simulink library "SUB_ECU_L4_MABX_HW_Interface"  (R2018a)
settings: Solver=VariableStepAuto  StartTime=0.0  StopTime=10.0  RelTol=1e-3
PostLoadFcn:
  | , if any(exist('dsrtsu_mdlpostloadfcn', 'file') == [2, 3, 6]), try dsrtsu_mdlpostloadfcn('Execute', bdroot); catch fprintf('Error in PostLoadFcn (dsrtsu_mdlpostloadfcn) for model "%s":\n %s\n', bdroot, lasterr); end, end,
undefined symbols (not defined in the file or in its folder): CANR_PROPB_REAX_3_13_CHANNEL_APV, CANR_PROPB_REAX_4_13_CHANNEL_APV, CANR_PROPB_XPR_1_50_CHANNEL_APV, ENUM_CAN_RX_T, ENUM_CAN_TX_T, ENUM_REAX_OPERATION_MODE_T, ENUM_SIGNAL_HEALTH_T, ENUM_XBR_CONTROL_MODE_T, ENUM_XBR_EBI_MODE_T, ENUM_XBR_PASS_THROUGH_ACTIVE_T, ENUM_XBR_PRIORITY_T, ENUM_XPR_INHIBIT_PARK_MANUAL_T, ENUM_XPR_INHIBIT_UNPARK_MANUAL_T, ENUM_XPR_PARK_MANUAL_T, ENUM_XPR_UNPARK_MANUAL_T, PROPB_REAX_1_E4_DES_POS_SIG_SRC_APV, PROPB_REAX_1_E4_DESIRED_OPMODE_APV, PROPB_REAX_1_E4_DESIRED_POSITION_APV, ptc_matlab_lib
libraries: PTC_MBDS_LIB x264, rtican x172, EmE_MBD_Blockset x39, simulink x34, $bdroot x16, rti1401lib_dio_type4 x8, simulink_need_slupdate x7, dsa_tcpip_lib x4, rti1401lib_adc_type4 x3, rtmapslib x3, rtitasklib x3
(part 13 of 51)

== system SUB_ECU_L4_MABX_HW_Interface/CAN_PIC_KW/CAN_RX_Bendix_RADAR_Tracks/RX_CAN_1 ==
  Enable : Inport
  Bus Creator : BusCreator  Inputs=74
  Data Type Conversion10 : DataTypeConversion  OutDataTypeStr=double  SaturateOnIntegerOverflow=on
  Data Type Conversion8 : DataTypeConversion  OutDataTypeStr=boolean  SaturateOnIntegerOverflow=on
  Data Type Conversion9 : DataTypeConversion  OutDataTypeStr=double  SaturateOnIntegerOverflow=on
  Tracks : rtican/RTICAN Receive (RX)   Reserved1=[]  Reserved2=[]  Reserved3=[]  Reserved4=[]  SfcnMessage=[]  Msg_Struct=[]  BoardTypeNo=[]  BoardNo=[]  ChannelNo=[]  Parameters=[]  DialogFcn=[]  UnitName=[]  Revision=[]  UnitValues=[]  DSProperties=struct('RTI',struct('Version',uint32(5),'BlockType',struct('isSLSource',uint8(1),'isSLSink',uint8(1),'isHWSource',uint8(0),'isHWSink',uint8(0),'isSetup',uint8(0),'isInline',uint8(1),'isNonInline',uint8(0),'isInterrupt',uint8(0),'isChannelwise',uint8(0)),'IOBoardType','RTICAN','UnitType','MESSAGE','Identifier','RX','DialogType','MSVC','BlockSet','RTICAN','SlaveProcessor','CAN'))  RTIBlockInterface=struct('OutputPortsWidth',int32([1 1 1 1 1 1 1 1 1 1 1 1 1 1 1 1 1 1 1 1 1 1 1 1 1 1 1 1 1 1 1 1 1 1 1 1 1 1 1 1 1 1 1 1 1 1 1 1 1 1 1 1 1 1 1 1 1 1 1 1 1 1 1 1 1 1 1 1 1 1 1 1 1 1]),'OutputPortsActive',ones(1,74),'OutputPortsName',{{'tr0_track_selection_status','tr0_corrected_lateral_distance','tr1_track_selection_status','tr1_corrected_lateral_distance','tr2_track_selection_status','tr2_corrected_lateral_distance','tr3_track_selection_status','tr3_corrected_lateral_distance','tr4_track_selection_status','tr4_corrected_lateral_distance','tr5_track_selection_status','tr5_corrected_lateral_distance','tr6_track_selection_status','tr6_corrected_lateral_distance','tr7_track_selection_status','tr7_corrected_lateral_distance','tr8_track_selection_status','tr8_corrected_lateral_distance','tr9_track_selection_status','tr9_corrected_lateral_distance','tr0_lateral_position','tr1_lateral_position','tr2_lateral_position','tr3_lateral_position','tr4_lateral_position','tr5_lateral_position','tr6_lateral_position','tr7_lateral_position','tr8_lateral_position','tr9_lateral_position','tr0_range','tr1_range','tr2_range','tr3_range','tr4_range','tr5_range','tr6_range','tr7_range','tr8_range','tr9_range','tr0_radar_confidence','tr1_radar_confidence','tr2_radar_confidence','tr3_radar_confidence','tr4_radar_confidence','tr5_radar_confidence','tr6_radar_confidence','tr7_radar_confidence','tr8_radar_confidence','tr9_radar_confidence','tr0_relative_velocitiy','tr0_acceleration_over_ground','tr1_relative_velocitiy','tr1_acceleration_over_ground','tr2_relative_velocitiy','tr2_acceleration_over_ground','tr3_relative_velocitiy','tr3_acceleration_over_ground','tr4_relative_velocitiy','tr4_acceleration_over_ground','tr5_relative_velocitiy','tr5_acceleration_over_ground','tr6_relative_velocitiy','tr6_acceleration_over_ground','tr7_relative_velocitiy','tr7_acceleration_over_ground','tr8_relative_velocitiy','tr8_acceleration_over_ground','tr9_relative_velocitiy','tr9_acceleration_over_ground','track_multiplexor',['RX status'],['RX time'],['RX delta time']}},'OutputPortsDataType',{{'SS_DOUBLE','SS_DOUBLE','SS_DOUBLE','SS_DOUBLE','SS_DOUBLE','SS_DOUBLE','SS_DOUBLE','SS_DOUBLE','SS_DOUBLE','SS_DOUBLE','SS_DOUBLE','SS_DOUBLE','SS_DOUBLE','SS_DOUBLE','SS_DOUBLE','SS_DOUBLE','SS_DOUBLE','SS_DOUBLE','SS_DOUBLE','SS_DOUBLE','SS_DOUBLE','SS_DOUBLE','SS_DOUBLE','SS_DOUBLE','SS_DOUBLE','SS_DOUBLE','SS_DOUBLE','SS_DOUBLE','SS_DOUBLE','SS_DOUBLE','SS_DOUBLE','SS_DOUBLE','SS_DOUBLE','SS_DOUBLE','SS_DOUBLE','SS_DOUBLE','SS_DOUBLE','SS_DOUBLE','SS_DOUBLE','SS_DOUBLE','SS_DOUBLE','SS_DOUBLE','SS_DOUBLE','SS_DOUBLE','SS_DOUBLE','SS_DOUBLE','SS_DOUBLE','SS_DOUBLE','SS_DOUBLE','SS_DOUBLE','SS_DOUBLE','SS_DOUBLE','SS_DOUBLE','SS_DOUBLE','SS_DOUBLE','SS_DOUBLE','SS_DOUBLE','SS_DOUBLE','SS_DOUBLE','SS_DOUBLE','SS_DOUBLE','SS_DOUBLE','SS_DOUBLE','SS_DOUBLE','SS_DOUBLE','SS_DOUBLE','SS_DOUBLE','SS_DOUBLE','SS_DOUBLE','SS_DOUBLE','SS_DOUBLE','SS_DOUBLE','SS_DOUBLE','SS_DOUBLE'}},'OutputPortsLabel',{{'tr0_track_selection_status','tr0_corrected_lateral_distance','tr1_track_selection_status','tr1_corrected_lateral_distance','tr2_track_selection_status','tr2_corrected_lateral_distance','tr3_track_selection_status','tr3_corrected_lateral_distance','tr4_track_selection_status','tr4_corrected_lateral_distance','tr5_track_selection_status','tr5_corrected_lateral_distance','tr6_track_selection_status','tr6_corrected_lateral_distance','tr7_track_selection_status','tr7_corrected_lateral_distance','tr8_track_selection_status','tr8_corrected_lateral_distance','tr9_track_selection_status','tr9_corrected_lateral_distance','tr0_lateral_position','tr1_lateral_position','tr2_lateral_position','tr3_lateral_position','tr4_lateral_position','tr5_lateral_position','tr6_lateral_position','tr7_lateral_position','tr8_lateral_position','tr9_lateral_position','tr0_range','tr1_range','tr2_range','tr3_range','tr4_range','tr5_range','tr6_range','tr7_range','tr8_range','tr9_range','tr0_radar_confidence','tr1_radar_confidence','tr2_radar_confidence','tr3_radar_confidence','tr4_radar_confidence','tr5_radar_confidence','tr6_radar_confidence','tr7_radar_confidence','tr8_radar_confidence','tr9_radar_confidence','tr0_relative_velocitiy','tr0_acceleration_over_ground','tr1_relative_velocitiy','tr1_acceleration_over_ground','tr2_relative_velocitiy','tr2_acceleration_over_ground','tr3_relative_velocitiy','tr3_acceleration_over_ground','tr4_relative_velocitiy','tr4_acceleration_over_ground','tr5_relative_velocitiy','tr5_acceleration_over_ground','tr6_relative_velocitiy','tr6_acceleration_over_ground','tr7_relative_velocitiy','tr7_acceleration_over_ground','tr8_relative_velocitiy','tr8_acceleration_over_ground','tr9_relative_velocitiy','tr9_acceleration_over_ground','track_multiplexor','','',''}},'OutputPortsLabelMode','ON','InputPortsWidth',int32(0),'InputPortsActive',0,'DialogFcn','rtican_message_interface_gui','BlockDisplay',{{'','center'}},'IconTransparency','on','ParameterTunableNames',{{}},'InitLevel',3,'BlockName',struct('Token',{{'Tracks'}}),'SampleTime',{{-1}},'TriggerPort',{{'none'}},'EnablePort',{{'yes'}})  RTIBlockParameters=struct('BoardTypeNo',{{1,'OFF',[]}},'BoardNo',{{2,'ON',[1 16]}},'ChannelNo',{{1,'ON',[1 2]}},'Parameters',{{struct('DataFileSupport',struct('DataFileSelectedMaster',1,'DataFileSelectedLocal',0,'DataFileName','c:\data\svn\truck1571\dbc\y257766_004_das_camera_objects_bendix_confidential.dbc|c:\data\svn\truck1571\dbc\y257766_004_das_radar_objects_bendix_confidential.dbc|','DataFileDate',{{{['31-Jan-2018 07:14:07']},{['31-Jan-2018 07:14:07']}}},'SelectedFile','dbc\y257766_004_das_radar_objects_bendix_confidential.dbc'),'Options',struct('StatusSelected',1,'TimeSelected',1,'DeltaTimeSelected',1,'BytePortSelected',0,'MessageLengthSelected',0,'TriggerPort',struct('Selected',0,'TriggerType',0),'UserCoding',struct('Selected',0,'InterfaceFile','UserDecodingFile','FcnName','UserDecodeFcn','InportSelected',0,'InportWidth',1,'OutportSelected',0,'OutportWidth',1),'EnablePortSelected',1,'SignalOnPortnameSelected',1,'UseRXService',1),'Message',struct('MsgOnBlocknameSelected',1,'MsgName','Tracks','MsgIdFormat',0,'MsgId',1635,'MsgLength',8,'NumSignals',71,'SampleTime',-1,'Signal',struct('SgnName',{'tr0_track_selection_status','tr0_corrected_lateral_distance','tr1_track_selection_status','tr1_corrected_lateral_distance','tr2_track_selection_status','tr2_corrected_lateral_distance','tr3_track_selection_status','tr3_corrected_lateral_distance','tr4_track_selection_status','tr4_corrected_lateral_distance','tr5_track_selection_status','tr5_corrected_lateral_distance','tr6_track_selection_status','tr6_corrected_lateral_distance','tr7_track_selection_status','tr7_corrected_lateral_distance','tr8_track_selection_status','tr8_corrected_lateral_distance','tr9_track_selection_status','tr9_corrected_lateral_distance','tr0_lateral_position','tr1_lateral_position','tr2_lateral_position','tr3_lateral_position','tr4_lateral_position','tr5_lateral_position','tr6_lateral_position','tr7_lateral_position','tr8_lateral_position','tr9_lateral_position','tr0_range','tr1_range','tr2_range','tr3_range','tr4_range','tr5_range','tr6_range','tr7_range','tr8_range','tr9_range','tr0_radar_confidence','tr1_radar_confidence','tr2_radar_confidence','tr3_radar_confidence','tr4_radar_confidence','tr5_radar_confidence','tr6_radar_confidence','tr7_radar_confidence','tr8_radar_confidence','tr9_radar_confidence','tr0_relative_velocitiy','tr0_acceleration_over_ground','tr1_relative_velocitiy','tr1_acceleration_over_ground','tr2_relative_velocitiy','tr2_acceleration_over_ground','tr3_relative_velocitiy','tr3_acceleration_over_ground','tr4_relative_velocitiy','tr4_acceleration_over_ground','tr5_relative_velocitiy','tr5_acceleration_over_ground','tr6_relative_velocitiy','tr6_acceleration_over_ground','tr7_relative_velocitiy','tr7_acceleration_over_ground','tr8_relative_velocitiy','tr8_acceleration_over_ground','tr9_relative_velocitiy','tr9_acceleration_over_ground','track_multiplexor'},'SgnStartBit',{0,0,0,0,0,0,0,0,0,0,0,0,0,0,0,0,0,0,0,0,14,14,14,14,14,14,14,14,14,14,16,16,16,16,16,16,16,16,16,16,24,24,24,24,24,24,24,24,24,24,32,32,32,32,32,32,32,32,32,32,32,32,32,32,32,32,32,32,32,32,56},'SgnLength',{13,16,13,16,13,16,13,16,13,16,13,16,13,16,13,16,13,16,13,16,10,10,10,10,10,10,10,10,10,10,16,16,16,16,16,16,16,16,16,16,8,8,8,8,8,8,8,8,8,8,14,8,14,8,14,8,14,8,14,8,14,8,14,8,14,8,14,8,14,8,8},'SgnType',{2,2,2,2,2,2,2,2,2,2,2,2,2,2,2,2,2,2,2,2,2,2,2,2,2,2,2,2,2,2,2,2,2,2,2,2,2,2,2,2,2,2,2,2,2,2,2,2,2,2,2,2,2,2,2,2,2,2,2,2,2,2,2,2,2,2,2,2,2,2,1},'ModeValue',{4,5,12,13,20,21,28,29,36,37,44,45,52,53,60,61,68,69,76,77,6,14,22,30,38,46,54,62,70,78,4,12,20,28,36,44,52,60,68,76,6,14,22,30,38,46,54,62,70,78,4,5,12,13,20,21,28,29,36,37,44,45,52,53,60,61,68,69,76,77,-1},'DataType',{0,1,0,1,0,1,0,1,0,1,0,1,0,1,0,1,0,1,0,1,1,1,1,1,1,1,1,1,1,1,0,0,0,0,0,0,0,0,0,0,0,0,0,0,0,0,0,0,0,0,1,0,1,0,1,0,1,0,1,0,1,0,1,0,1,0,1,0,1,0,0},'ByteLayout',{2,2,2,2,2,2,2,2,2,2,2,2,2,2,2,2,2,2,2,2,2,2,2,2,2,2,2,2,2,2,2,2,2,2,2,2,2,2,2,2,2,2,2,2,2,2,2,2,2,2,2,2,2,2,2,2,2,2,2,2,2,2,2,2,2,2,2,2,2,2,2},'Factor',{1,0.001,1,0.001,1,0.001,1,0.001,1,0.001,1,0.001,1,0.001,1,0.001,1,0.001,1,0.001,0.1,0.1,0.1,0.1,0.1,0.1,0.1,0.1,0.1,0.1,0.01,0.01,0.01,0.01,0.01,0.01,0.01,0.01,0.01,0.01,0.0039215686274509803,0.0039215686274509803,0.0039215686274509803,0.0039215686274509803,0.0039215686274509803,0.0039215686274509803,0.0039215686274509803,0.0039215686274509803,0.0039215686274509803,0.0039215686274509803,0.01,0.05,0.01,0.05,0.01,0.05,0.01,0.05,0.01,0.05,0.01,0.05,0.01,0.05,0.01,0.05,0.01,0.05,0.01,0.05,1},'Offset',{0,0,0,0,0,0,0,0,0,0,0,0,0,0,0,0,0,0,0,0,0,0,0,0,0,0,0,0,0,0,0,0,0,0,0,0,0,0,0,0,0,0,0,0,0,0,0,0,0,0,0,-8.8,0,-8.8,0,-8.8,0,-8.8,0,-8.8,0,-8.8,0,-8.8,0,-8.8,0,-8.8,0,-8.8,0},'SgnComment',{{''},{''},{''},{''},{''},{''},{''},{''},{''},{''},{''},{''},{''},{''},{''},{''},{''},{''},{''},{''},{''},{''},{''},{''},{''},{''},{''},{''},{''},{''},{''},{''},{''},{''},{''},{''},{''},{''},{''},{''},{''},{''},{''},{''},{''},{''},{''},{''},{''},{''},{''},{''},{''},{''},{''},{''},{''},{''},{''},{''},{''},{''},{''},{''},{''},{''},{''},{''},{''},{''},{''}},'SgnUnit',{'','m','','m','','m','','m','','m','','m','','m','','m','','m','','m','m','m','m','m','m','m','m','m','m','m','m','m','m','m','m','m','m','m','m','m','','','','','','','','','','','m/s','m/s²','m/s','m/s²','m/s','m/s²','m/s','m/s²','m/s','m/s²','m/s','m/s²','m/s','m/s²','m/s','m/s²','m/s','m/s²','m/s','m/s²',''},'Min',{0,0,0,0,0,0,0,0,0,0,0,0,0,0,0,0,0,0,0,0,0,0,0,0,0,0,0,0,0,0,0,0,0,0,0,0,0,0,0,0,0,0,0,0,0,0,0,0,0,0,0,0,0,0,0,0,0,0,0,0,0,0,0,0,0,0,0,0,0,0,0},'Max',{0,0,0,0,0,0,0,0,0,0,0,0,0,0,0,0,0,0,0,0,0,0,0,0,0,0,0,0,0,0,0,0,0,0,0,0,0,0,0,0,1,1,1,1,1,1,1,1,1,1,0,0,0,0,0,0,0,0,0,0,0,0,0,0,0,0,0,0,0,0,0},'SLDataType',{'SS_DOUBLE','SS_DOUBLE','SS_DOUBLE','SS_DOUBLE','SS_DOUBLE','SS_DOUBLE','SS_DOUBLE','SS_DOUBLE','SS_DOUBLE','SS_DOUBLE','SS_DOUBLE','SS_DOUBLE','SS_DOUBLE','SS_DOUBLE','SS_DOUBLE','SS_DOUBLE','SS_DOUBLE','SS_DOUBLE','SS_DOUBLE','SS_DOUBLE','SS_DOUBLE','SS_DOUBLE','SS_DOUBLE','SS_DOUBLE','SS_DOUBLE','SS_DOUBLE','SS_DOUBLE','SS_DOUBLE','SS_DOUBLE','SS_DOUBLE','SS_DOUBLE','SS_DOUBLE','SS_DOUBLE','SS_DOUBLE','SS_DOUBLE','SS_DOUBLE','SS_DOUBLE','SS_DOUBLE','SS_DOUBLE','SS_DOUBLE','SS_DOUBLE','SS_DOUBLE','SS_DOUBLE','SS_DOUBLE','SS_DOUBLE','SS_DOUBLE','SS_DOUBLE','SS_DOUBLE','SS_DOUBLE','SS_DOUBLE','SS_DOUBLE','SS_DOUBLE','SS_DOUBLE','SS_DOUBLE','SS_DOUBLE','SS_DOUBLE','SS_DOUBLE','SS_DOUBLE','SS_DOUBLE','SS_DOUBLE','SS_DOUBLE','SS_DOUBLE','SS_DOUBLE','SS_DOUBLE','SS_DOUBLE','SS_DOUBLE','SS_DOUBLE','SS_DOUBLE','SS_DOUBLE','SS_DOUBLE','SS_DOUBLE'}),'MsgIdNumFormat',1,'MsgComment',{{''}}),'Version',1.2,'general',struct('isFromLib',0)),'OFF',[]}},'GroupId',{{struct('Group',{{'RTICAN'}},'No',27,'Behavior',{{'NAMECHANGE'}},'BlockType',{{'SINK'}},'NameChangeFlag',0),'OFF',[]}},'SFcnRTICANMessage',{{struct('MsgType','RX','SFcnPortType','Scalar','MsgName','Tracks','MsgIdFormat','STD','MsgId',1635,'MsgLength',8,'NumSignals',71,'SampleTime',-1,'Signal',struct('SgnName',{'tr0_track_selection_status','tr0_corrected_lateral_distance','tr1_track_selection_status','tr1_corrected_lateral_distance','tr2_track_selection_status','tr2_corrected_lateral_distance','tr3_track_selection_status','tr3_corrected_lateral_distance','tr4_track_selection_status','tr4_corrected_lateral_distance','tr5_track_selection_status','tr5_corrected_lateral_distance','tr6_track_selection_status','tr6_corrected_lateral_distance','tr7_track_selection_status','tr7_corrected_lateral_distance','tr8_track_selection_status','tr8_corrected_lateral_distance','tr9_track_selection_status','tr9_corrected_lateral_distance','tr0_lateral_position','tr1_lateral_position','tr2_lateral_position','tr3_lateral_position','tr4_lateral_position','tr5_lateral_position','tr6_lateral_position','tr7_lateral_position','tr8_lateral_position','tr9_lateral_position','tr0_range','tr1_range','tr2_range','tr3_range','tr4_range','tr5_range','tr6_range','tr7_range','tr8_range','tr9_range','tr0_radar_confidence','tr1_radar_confidence','tr2_radar_confidence','tr3_radar_confidence','tr4_radar_confidence','tr5_radar_confidence','tr6_radar_confidence','tr7_radar_confidence','tr8_radar_confidence','tr9_radar_confidence','tr0_relative_velocitiy','tr0_acceleration_over_ground','tr1_relative_velocitiy','tr1_acceleration_over_ground','tr2_relative_velocitiy','tr2_acceleration_over_ground','tr3_relative_velocitiy','tr3_acceleration_over_ground','tr4_relative_velocitiy','tr4_acceleration_over_ground','tr5_relative_velocitiy','tr5_acceleration_over_ground','tr6_relative_velocitiy','tr6_acceleration_over_ground','tr7_relative_velocitiy','tr7_acceleration_over_ground','tr8_relative_velocitiy','tr8_acceleration_over_ground','tr9_relative_velocitiy','tr9_acceleration_over_ground','track_multiplexor'},'SgnStartBit',{0,0,0,0,0,0,0,0,0,0,0,0,0,0,0,0,0,0,0,0,14,14,14,14,14,14,14,14,14,14,16,16,16,16,16,16,16,16,16,16,24,24,24,24,24,24,24,24,24,24,32,32,32,32,32,32,32,32,32,32,32,32,32,32,32,32,32,32,32,32,56},'SgnLength',{13,16,13,16,13,16,13,16,13,16,13,16,13,16,13,16,13,16,13,16,10,10,10,10,10,10,10,10,10,10,16,16,16,16,16,16,16,16,16,16,8,8,8,8,8,8,8,8,8,8,14,8,14,8,14,8,14,8,14,8,14,8,14,8,14,8,14,8,14,8,8},'SgnType',{'mode-dependent','mode-dependent','mode-dependent','mode-dependent','mode-dependent','mode-dependent','mode-dependent','mode-dependent','mode-dependent','mode-dependent','mode-dependent','mode-dependent','mode-dependent','mode-dependent','mode-dependent','mode-dependent','mode-dependent','mode-dependent','mode-dependent','mode-dependent','mode-dependent','mode-dependent','mode-dependent','mode-dependent','mode-dependent','mode-dependent','mode-dependent','mode-dependent','mode-dependent','mode-dependent','mode-dependent','mode-dependent','mode-dependent','mode-dependent','mode-dependent','mode-dependent','mode-dependent','mode-dependent','mode-dependent','mode-dependent','mode-dependent','mode-dependent','mode-dependent','mode-dependent','mode-dependent','mode-dependent','mode-dependent','mode-dependent','mode-dependent','mode-dependent','mode-dependent','mode-dependent','mode-dependent','mode-dependent','mode-dependent','mode-dependent','mode-dependent','mode-dependent','mode-dependent','mode-dependent','mode-dependent','mode-dependent','mode-dependent','mode-dependent','mode-dependent','mode-dependent','mode-dependent','mode-dependent','mode-dependent','mode-dependent','mode'},'ModeValue',{4,5,12,13,20,21,28,29,36,37,44,45,52,53,60,61,68,69,76,77,6,14,22,30,38,46,54,62,70,78,4,12,20,28,36,44,52,60,68,76,6,14,22,30,38,46,54,62,70,78,4,5,12,13,20,21,28,29,36,37,44,45,52,53,60,61,68,69,76,77,-1},'DataType',{['unsigned int'],['signed int'],['unsigned int'],['signed int'],['unsigned int'],['signed int'],['unsigned int'],['signed int'],['unsigned int'],['signed int'],['unsigned int'],['signed int'],['unsigned int'],['signed int'],['unsigned int'],['signed int'],['unsigned int'],['signed int'],['unsigned int'],['signed int'],['signed int'],['signed int'],['signed int'],['signed int'],['signed int'],['signed int'],['signed int'],['signed int'],['signed int'],['signed int'],['unsigned int'],['unsigned int'],['unsigned int'],['unsigned int'],['unsigned int'],['unsigned int'],['unsigned int'],['unsigned int'],['unsigned int'],['unsigned int'],['unsigned int'],['unsigned int'],['unsigned int'],['unsigned int'],['unsigned int'],['unsigned int'],['unsigned int'],['unsigned int'],['unsigned int'],['unsigned int'],['signed int'],['unsigned int'],['signed int'],['unsigned int'],['signed int'],['unsigned int'],['signed int'],['unsigned int'],['signed int'],['unsigned int'],['signed int'],['unsigned int'],['signed int'],['unsigned int'],['signed int'],['unsigned int'],['signed int'],['unsigned int'],['signed int'],['unsigned int'],['unsigned int']},'ByteLayout',{['motorola back.'],['motorola back.'],['motorola back.'],['motorola back.'],['motorola back.'],['motorola back.'],['motorola back.'],['motorola back.'],['motorola back.'],['motorola back.'],['motorola back.'],['motorola back.'],['motorola back.'],['motorola back.'],['motorola back.'],['motorola back.'],['motorola back.'],['motorola back.'],['motorola back.'],['motorola back.'],['motorola back.'],['motorola back.'],['motorola back.'],['motorola back.'],['motorola back.'],['motorola back.'],['motorola back.'],['motorola back.'],['motorola back.'],['motorola back.'],['motorola back.'],['motorola back.'],['motorola back.'],['motorola back.'],['motorola back.'],['motorola back.'],['motorola back.'],['motorola back.'],['motorola back.'],['motorola back.'],['motorola back.'],['motorola back.'],['motorola back.'],['motorola back.'],['motorola back.'],['motorola back.'],['motorola back.'],['motorola back.'],['motorola back.'],['motorola back.'],['motorola back.'],['motorola back.'],['motorola back.'],['motorola back.'],['motorola back.'],['motorola back.'],['motorola back.'],['motorola back.'],['motorola back.'],['motorola back.'],['motorola back.'],['motorola back.'],['motorola back.'],['motorola back.'],['motorola back.'],['motorola back.'],['motorola back.'],['motorola back.'],['motorola back.'],['motorola back.'],['motorola back.']},'Factor',{1,0.001,1,0.001,1,0.001,1,0.001,1,0.001,1,0.001,1,0.001,1,0.001,1,0.001,1,0.001,0.1,0.1,0.1,0.1,0.1,0.1,0.1,0.1,0.1,0.1,0.01,0.01,0.01,0.01,0.01,0.01,0.01,0.01,0.01,0.01,0.0039215686274509803,0.0039215686274509803,0.0039215686274509803,0.0039215686274509803,0.0039215686274509803,0.0039215686274509803,0.0039215686274509803,0.0039215686274509803,0.0039215686274509803,0.0039215686274509803,0.01,0.05,0.01,0.05,0.01,0.05,0.01,0.05,0.01,0.05,0.01,0.05,0.01,0.05,0.01,0.05,0.01,0.05,0.01,0.05,1},'Offset',{0,0,0,0,0,0,0,0,0,0,0,0,0,0,0,0,0,0,0,0,0,0,0,0,0,0,0,0,0,0,0,0,0,0,0,0,0,0,0,0,0,0,0,0,0,0,0,0,0,0,0,-8.8,0,-8.8,0,-8.8,0,-8.8,0,-8.8,0,-8.8,0,-8.8,0,-8.8,0,-8.8,0,-8.8,0},'SLDataType',{'SS_DOUBLE','SS_DOUBLE','SS_DOUBLE','SS_DOUBLE','SS_DOUBLE','SS_DOUBLE','SS_DOUBLE','SS_DOUBLE','SS_DOUBLE','SS_DOUBLE','SS_DOUBLE','SS_DOUBLE','SS_DOUBLE','SS_DOUBLE','SS_DOUBLE','SS_DOUBLE','SS_DOUBLE','SS_DOUBLE','SS_DOUBLE','SS_DOUBLE','SS_DOUBLE','SS_DOUBLE','SS_DOUBLE','SS_DOUBLE','SS_DOUBLE','SS_DOUBLE','SS_DOUBLE','SS_DOUBLE','SS_DOUBLE','SS_DOUBLE','SS_DOUBLE','SS_DOUBLE','SS_DOUBLE','SS_DOUBLE','SS_DOUBLE','SS_DOUBLE','SS_DOUBLE','SS_DOUBLE','SS_DOUBLE','SS_DOUBLE','SS_DOUBLE','SS_DOUBLE','SS_DOUBLE','SS_DOUBLE','SS_DOUBLE','SS_DOUBLE','SS_DOUBLE','SS_DOUBLE','SS_DOUBLE','SS_DOUBLE','SS_DOUBLE','SS_DOUBLE','SS_DOUBLE','SS_DOUBLE','SS_DOUBLE','SS_DOUBLE','SS_DOUBLE','SS_DOUBLE','SS_DOUBLE','SS_DOUBLE','SS_DOUBLE','SS_DOUBLE','SS_DOUBLE','SS_DOUBLE','SS_DOUBLE','SS_DOUBLE','SS_DOUBLE','SS_DOUBLE','SS_DOUBLE','SS_DOUBLE','SS_DOUBLE'}),'StatusSelected','yes','TimeSelected','yes','DeltaTimeSelected','yes','BytePortSelected','no','MessageLengthSelected','no','TriggerPort',struct('Selected','no','TriggerType',0),'UserCoding',struct('Selected','no','InterfaceFile','UserDecodingFile','FcnName','UserDecodeFcn','InportSelected','no','InportWidth',1,'OutportSelected','no','OutportWidth',1),'EnablePortSelected','yes','UseRXService','yes','BoardType','DS1','BoardNo',2,'ControllerNo',1),'OFF',[]}},'TLCFileName',{{'rtican_rx_message','OFF',[]}})  RTISFcnParameters=struct('SFcnRTICANMessage','struct','TLCFileName','char')  RTIBlockParaDefault=struct('BoardTypeNo',4302,'BoardNo',1,'ChannelNo',1,'Parameters',struct('DataFileSupport',struct('DataFileSelectedMaster',0,'DataFileSelectedLocal',0,'DataFileName','','DataFileDate','','SelectedFile',['<no file selected>']),'Options',struct('StatusSelected',1,'TimeSelected',1,'DeltaTimeSelected',1,'BytePortSelected',0,'MessageLengthSelected',0,'TriggerPort',struct('Selected',0,'TriggerType','rising'),'UserCoding',struct('Selected',0,'InterfaceFile','UserDecodingFile','FcnName','UserDecodeFcn','InportSelected',0,'InportWidth',1,'OutportSelected',0,'OutportWidth',1),'EnablePortSelected',0,'SignalOnPortnameSelected',1,'UseRXService',0),'Message',struct('MsgOnBlocknameSelected',0,'MsgName',['RX Message'],'MsgIdFormat',0,'MsgId',100,'MsgLength',8,'NumSignals',1,'SampleTime',-1,'Signal',struct('SgnName',['RX signal'],'SgnStartBit',0,'SgnLength',8,'SgnType',0,'ModeValue',-1,'DataType',0,'SLDataType','SS_DOUBLE','ByteLayout',0,'Factor',1,'Offset',0,'Min',0,'Max',255,'SgnComment',{{}},'SgnUnit',''),'MsgIdNumFormat',0,'MsgComment',{{''}}),'Version',1.2,'general',struct('isFromLib',1)),'GroupId',struct('Group',{{'RTICAN'}},'No',1,'Behavior',{{'NAMECHANGE'}},'BlockType',{{'SINK'}},'NameChangeFlag',0),'SFcnRTICANMessage',struct('MsgType','RX','MsgName',['RX Message'],'MsgIdFormat','STD','MsgId',100,'MsgLength',8,'NumSignals',1,'SampleTime',-1,'Signal',struct('SgnName',['RX signal'],'SgnStartBit',0,'SgnLength',8,'SgnType','standard','ModeValue',-1,'DataType',['unsigned int'],'ByteLayout',['little endian'],'SLDataType','SS_DOUBLE','Factor',1,'Offset',0),'StatusSelected','yes','TimeSelected','yes','DeltaTimeSelected','yes','BytePortSelected','no','MessageLengthSelected','no','EnablePortSelected','no','UserCoding',struct('Selected','no','InterfaceFile','UserDecodingFile','FcnName','UserDecodeFcn','InportSelected','no','InportWidth',1,'OutportSelected','no','OutportWidth',1),'TriggerPort',struct('Selected','no','TriggerType','rising'),'UseRXService','no','BoardType','DS4302','BoardNo',1,'ControllerNo',1,'SFcnPortType','Scalar'),'TLCFileName','rtican_rx_message')
      settings: AttributesFormatString=Group Id: RTICAN27\n  SourceProductName=dSPACE RTI CAN Blockset
  Bendix_RADAR_Tracks : Outport
  wires:
  Enable/1 -> Tracks/Enable
  Tracks/74 -> Data Type Conversion10/1
  Tracks/73 -> Data Type Conversion9/1
  Tracks/72 -> Data Type Conversion8/1
  Tracks/29 -> Bus Creator/29  "tr8_lateral_position"
  Tracks/28 -> Bus Creator/28  "tr7_lateral_position"
  Tracks/30 -> Bus Creator/30  "tr9_lateral_position"
  Tracks/27 -> Bus Creator/27  "tr6_lateral_position"
  Tracks/31 -> Bus Creator/31  "tr0_range"
  Tracks/26 -> Bus Creator/26  "tr5_lateral_position"
  Tracks/32 -> Bus Creator/32  "tr1_range"
  Tracks/25 -> Bus Creator/25  "tr4_lateral_position"
  Tracks/33 -> Bus Creator/33  "tr2_range"
  Tracks/24 -> Bus Creator/24  "tr3_lateral_position"
  Tracks/34 -> Bus Creator/34  "tr3_range"
  Tracks/23 -> Bus Creator/23  "tr2_lateral_position"
  Tracks/35 -> Bus Creator/35  "tr4_range"
  Tracks/22 -> Bus Creator/22  "tr1_lateral_position"
  Tracks/36 -> Bus Creator/36  "tr5_range"
  Tracks/21 -> Bus Creator/21  "tr0_lateral_position"
  Tracks/37 -> Bus Creator/37  "tr6_range"
  Tracks/20 -> Bus Creator/20  "tr9_corrected_lateral_distance"
  Tracks/38 -> Bus Creator/38  "tr7_range"
  Tracks/19 -> Bus Creator/19  "tr9_track_selection_status"
  Tracks/39 -> Bus Creator/39  "tr8_range"
  Tracks/18 -> Bus Creator/18  "tr8_corrected_lateral_distance"
  Tracks/40 -> Bus Creator/40  "tr9_range"
  Tracks/17 -> Bus Creator/17  "tr8_track_selection_status"
  Tracks/41 -> Bus Creator/41  "tr0_radar_confidence"
  Tracks/16 -> Bus Creator/16  "tr7_corrected_lateral_distance"
  Tracks/42 -> Bus Creator/42  "tr1_radar_confidence"
  Tracks/15 -> Bus Creator/15  "tr7_track_selection_status"
  Tracks/43 -> Bus Creator/43  "tr2_radar_confidence"
  Tracks/14 -> Bus Creator/14  "tr6_corrected_lateral_distance"
  Tracks/44 -> Bus Creator/44  "tr3_radar_confidence"
  Tracks/13 -> Bus Creator/13  "tr6_track_selection_status"
  Tracks/45 -> Bus Creator/45  "tr4_radar_confidence"
  Tracks/12 -> Bus Creator/12  "tr5_corrected_lateral_distance"
  Tracks/46 -> Bus Creator/46  "tr5_radar_confidence"
  Tracks/11 -> Bus Creator/11  "tr5_track_selection_status"
  Tracks/47 -> Bus Creator/47  "tr6_radar_confidence"
  Tracks/10 -> Bus Creator/10  "tr4_corrected_lateral_distance"
  Tracks/48 -> Bus Creator/48  "tr7_radar_confidence"
  Tracks/9 -> Bus Creator/9  "tr4_track_selection_status"
  Tracks/49 -> Bus Creator/49  "tr8_radar_confidence"
  Tracks/8 -> Bus Creator/8  "tr3_corrected_lateral_distance"
  Tracks/50 -> Bus Creator/50  "tr9_radar_confidence"
  Tracks/7 -> Bus Creator/7  "tr3_track_selection_status"
  Tracks/51 -> Bus Creator/51  "tr0_relative_velocitiy"
  Tracks/6 -> Bus Creator/6  "tr2_corrected_lateral_distance"
  Tracks/52 -> Bus Creator/52  "tr0_acceleration_over_ground"
  Tracks/5 -> Bus Creator/5  "tr2_track_selection_status"
  Tracks/53 -> Bus Creator/53  "tr1_relative_velocitiy"
  Tracks/4 -> Bus Creator/4  "tr1_corrected_lateral_distance"
  Tracks/54 -> Bus Creator/54  "tr1_acceleration_over_ground"
  Tracks/3 -> Bus Creator/3  "tr1_track_selection_status"
  Tracks/55 -> Bus Creator/55  "tr2_relative_velocitiy"
  Tracks/2 -> Bus Creator/2  "tr0_corrected_lateral_distance"
  Tracks/56 -> Bus Creator/56  "tr2_acceleration_over_ground"
  Tracks/1 -> Bus Creator/1  "tr0_track_selection_status"
  Tracks/57 -> Bus Creator/57  "tr3_relative_velocitiy"
  Tracks/58 -> Bus Creator/58  "tr3_acceleration_over_ground"
  Tracks/59 -> Bus Creator/59  "tr4_relative_velocitiy"
  Tracks/60 -> Bus Creator/60  "tr4_acceleration_over_ground"
  Tracks/61 -> Bus Creator/61  "tr5_relative_velocitiy"
  Tracks/62 -> Bus Creator/62  "tr5_acceleration_over_ground"
  Tracks/63 -> Bus Creator/63  "tr6_relative_velocitiy"
  Tracks/64 -> Bus Creator/64  "tr6_acceleration_over_ground"
  Tracks/65 -> Bus Creator/65  "tr7_relative_velocitiy"
  Tracks/66 -> Bus Creator/66  "tr7_acceleration_over_ground"
  Tracks/67 -> Bus Creator/67  "tr8_relative_velocitiy"
  Tracks/68 -> Bus Creator/68  "tr8_acceleration_over_ground"
  Tracks/69 -> Bus Creator/69  "tr9_relative_velocitiy"
  Tracks/70 -> Bus Creator/70  "tr9_acceleration_over_ground"
  Tracks/71 -> Bus Creator/71  "track_multiplexor"
  Data Type Conversion8/1 -> Bus Creator/72  "Bendix_RADAR_Tracks_RX_status"
  Data Type Conversion9/1 -> Bus Creator/73  "Bendix_RADAR_Tracks_RX_time"
  Data Type Conversion10/1 -> Bus Creator/74  "Bendix_RADAR_Tracks_RX_delta_time"
  Bus Creator/1 -> Bendix_RADAR_Tracks/1  "Bendix_RADAR_Tracks"

== system SUB_ECU_L4_MABX_HW_Interface/CAN_PIC_KW/CAN_RX_CCVS1_00/RX_CAN_1 ==
  Enable : Inport
  Bus Creator : BusCreator  Inputs=20
  Bus Creator3 : BusCreator  Inputs=4
  CCVS1_00 : rtican/RTICAN Receive (RX)   Reserved1=[]  Reserved2=[]  Reserved3=[]  Reserved4=[]  SfcnMessage=[]  Msg_Struct=[]  BoardTypeNo=[]  BoardNo=[]  ChannelNo=[]  Parameters=[]  DialogFcn=[]  UnitName=[]  Revision=[]  UnitValues=[]  DSProperties=struct('RTI',struct('Version',uint32(5),'BlockType',struct('isSLSource',uint8(1),'isSLSink',uint8(1),'isHWSource',uint8(0),'isHWSink',uint8(0),'isSetup',uint8(0),'isInline',uint8(1),'isNonInline',uint8(0),'isInterrupt',uint8(0),'isChannelwise',uint8(0)),'IOBoardType','RTICAN','UnitType','MESSAGE','Identifier','RX','DialogType','MSVC','BlockSet','RTICAN','SlaveProcessor','CAN'))  RTIBlockInterface=struct('OutputPortsWidth',int32([1 1 1 1 1 1 1 1 1 1 1 1 1 1 1 1 1 1 1 1 1 1 1]),'OutputPortsActive',ones(1,23),'OutputPortsName',{{'TwoSpeedAxleSwitch','ParkingBrakeSwitch','CruiseCtrlPauseSwitch','ParkBrakeReleaseInhibitRq','WheelBasedVehicleSpeed','CruiseCtrlActive','CruiseCtrlEnableSwitch','BrakeSwitch','ClutchSwitch','CruiseCtrlSetSwitch','CruiseCtrlCoastSwitch','CruiseCtrlResumeSwitch','CruiseCtrlAccelerateSwitch','CruiseCtrlSetSpeed','PTOGovernorState','CruiseCtrlStates','EngIdleIncrementSwitch','EngIdleDecrementSwitch','EngTestModeSwitch','EngShutdownOverrideSwitch',['RX status'],['RX time'],['RX delta time']}},'OutputPortsDataType',{{'SS_DOUBLE','SS_DOUBLE','SS_DOUBLE','SS_DOUBLE','SS_DOUBLE','SS_DOUBLE','SS_DOUBLE','SS_DOUBLE','SS_DOUBLE','SS_DOUBLE','SS_DOUBLE','SS_DOUBLE','SS_DOUBLE','SS_DOUBLE','SS_DOUBLE','SS_DOUBLE','SS_DOUBLE','SS_DOUBLE','SS_DOUBLE','SS_DOUBLE','SS_DOUBLE','SS_DOUBLE','SS_DOUBLE'}},'OutputPortsLabel',{{'TwoSpeedAxleSwitch','ParkingBrakeSwitch','CruiseCtrlPauseSwitch','ParkBrakeReleaseInhibitRq','WheelBasedVehicleSpeed','CruiseCtrlActive','CruiseCtrlEnableSwitch','BrakeSwitch','ClutchSwitch','CruiseCtrlSetSwitch','CruiseCtrlCoastSwitch','CruiseCtrlResumeSwitch','CruiseCtrlAccelerateSwitch','CruiseCtrlSetSpeed','PTOGovernorState','CruiseCtrlStates','EngIdleIncrementSwitch','EngIdleDecrementSwitch','EngTestModeSwitch','EngShutdownOverrideSwitch','','',''}},'OutputPortsLabelMode','ON','InputPortsWidth',int32(0),'InputPortsActive',0,'DialogFcn','rtican_message_interface_gui','BlockDisplay',{{'','center'}},'IconTransparency','on','ParameterTunableNames',{{}},'InitLevel',3,'BlockName',struct('Token',{{'CCVS1_00'}}),'SampleTime',{{-1}},'TriggerPort',{{'none'}},'EnablePort',{{'yes'}})  RTIBlockParameters=struct('BoardTypeNo',{{1,'OFF',[]}},'BoardNo',{{1,'ON',[1 16]}},'ChannelNo',{{1,'ON',[1 2]}},'Parameters',{{struct('DataFileSupport',struct('DataFileSelectedMaster',1,'DataFileSelectedLocal',0,'DataFileName','c:\localdata\chris\advanced_tech\adas\level4_rcp\truck1571\dbc\mabx_can1.dbc|','DataFileDate',{{{['03-Apr-2017 12:55:40']}}},'SelectedFile',['<no file selected>']),'Options',struct('StatusSelected',1,'TimeSelected',1,'DeltaTimeSelected',1,'BytePortSelected',0,'MessageLengthSelected',0,'TriggerPort',struct('Selected',0,'TriggerType',0),'UserCoding',struct('Selected',0,'InterfaceFile','UserDecodingFile','FcnName','UserDecodeFcn','InportSelected',0,'InportWidth',1,'OutportSelected',0,'OutportWidth',1),'EnablePortSelected',1,'SignalOnPortnameSelected',1,'UseRXService',1),'Message',struct('MsgOnBlocknameSelected',1,'MsgName','CCVS1_00','MsgIdFormat',1,'MsgId',218034432,'MsgLength',8,'NumSignals',20,'SampleTime',-1,'Signal',struct('SgnName',{'TwoSpeedAxleSwitch','ParkingBrakeSwitch','CruiseCtrlPauseSwitch','ParkBrakeReleaseInhibitRq','WheelBasedVehicleSpeed','CruiseCtrlActive','CruiseCtrlEnableSwitch','BrakeSwitch','ClutchSwitch','CruiseCtrlSetSwitch','CruiseCtrlCoastSwitch','CruiseCtrlResumeSwitch','CruiseCtrlAccelerateSwitch','CruiseCtrlSetSpeed','PTOGovernorState','CruiseCtrlStates','EngIdleIncrementSwitch','EngIdleDecrementSwitch','EngTestModeSwitch','EngShutdownOverrideSwitch'},'SgnStartBit',{0,2,4,6,8,24,26,28,30,32,34,36,38,40,48,53,56,58,60,62},'SgnLength',{2,2,2,2,16,2,2,2,2,2,2,2,2,8,5,3,2,2,2,2},'SgnType',{0,0,0,0,0,0,0,0,0,0,0,0,0,0,0,0,0,0,0,0},'ModeValue',{-1,-1,-1,-1,-1,-1,-1,-1,-1,-1,-1,-1,-1,-1,-1,-1,-1,-1,-1,-1},'DataType',{0,0,0,0,0,0,0,0,0,0,0,0,0,0,0,0,0,0,0,0},'ByteLayout',{0,0,0,0,0,0,0,0,0,0,0,0,0,0,0,0,0,0,0,0},'Factor',{1,1,1,1,2^-8,1,1,1,1,1,1,1,1,1,1,1,1,1,1,1},'Offset',{0,0,0,0,0,0,0,0,0,0,0,0,0,0,0,0,0,0,0,0},'SgnComment',{{['Switch signal which indicates the current axle range.']},{['Switch signal which indicates when the parking brake is set.']},{['Switch signal which indicates the position of the Cruise Control Pause Switch used on Remote Cruise Control applications.']},{['Park Brake Release Inhibit Request signals the desire that an applied park brake remain applied and limit the ability of the']},{['Speed of the vehicle as calculated from wheel or tailshaft speed.']},{['Cruise control is switched on.']},{['Switch signal which indicates that it is possible to manage the cruise control function.']},{['Switch signal which indicates that the driver operated brake foot pedal is being pressed.']},{['Switch signal which indicates that the clutch pedal is being pressed.']},{['Switch signal of the cruise control activator which indicates that the activator is in the position “set.']},{['Switch signal of the cruise control activator which indicates that the activator is in the position “coast (decelerate).']},{['Switch signal of the cruise control activator which indicates that the activator is in the position “resume.']},{['Switch signal of the cruise control activator which indicates that the activator is in the position “accelerate.']},{['Value of set (chosen) velocity of velocity control system.']},{['This parameter is used to indicate the current state or mode of operation by the power takeoff (PTO) governor.']},{['This parameter is used to indicate the current state, or mode, of operation by the cruise control device.']},{['Switch signal which indicates the position of the idle increment switch.']},{['Switch signal which indicates the position of the idle decrement switch.']},{['Switch signal which indicates the position of the engine test mode switch.']},{['Switch signal which indicates the position of the engine shutdown override switch.']}},'SgnUnit',{'','','','','km/h','','','','','','','','','km/h','','','','','',''},'Min',{0,0,0,0,0,0,0,0,0,0,0,0,0,0,0,0,0,0,0,0},'Max',{3,3,3,3,250.996,3,3,3,3,3,3,3,3,250,31,7,3,3,3,3},'SLDataType',{'SS_DOUBLE','SS_DOUBLE','SS_DOUBLE','SS_DOUBLE','SS_DOUBLE','SS_DOUBLE','SS_DOUBLE','SS_DOUBLE','SS_DOUBLE','SS_DOUBLE','SS_DOUBLE','SS_DOUBLE','SS_DOUBLE','SS_DOUBLE','SS_DOUBLE','SS_DOUBLE','SS_DOUBLE','SS_DOUBLE','SS_DOUBLE','SS_DOUBLE'}),'MsgIdNumFormat',1,'MsgComment',{{['Cruise Control/Vehicle Speed']}}),'Version',1.2,'general',struct('isFromLib',0)),'OFF',[]}},'GroupId',{{struct('Group',{{'RTICAN'}},'No',25,'Behavior',{{'NAMECHANGE'}},'BlockType',{{'SINK'}},'NameChangeFlag',0),'OFF',[]}},'SFcnRTICANMessage',{{struct('MsgType','RX','SFcnPortType','Scalar','MsgName','CCVS1_00','MsgIdFormat','XTD','MsgId',218034432,'MsgLength',8,'NumSignals',20,'SampleTime',-1,'Signal',struct('SgnName',{'TwoSpeedAxleSwitch','ParkingBrakeSwitch','CruiseCtrlPauseSwitch','ParkBrakeReleaseInhibitRq','WheelBasedVehicleSpeed','CruiseCtrlActive','CruiseCtrlEnableSwitch','BrakeSwitch','ClutchSwitch','CruiseCtrlSetSwitch','CruiseCtrlCoastSwitch','CruiseCtrlResumeSwitch','CruiseCtrlAccelerateSwitch','CruiseCtrlSetSpeed','PTOGovernorState','CruiseCtrlStates','EngIdleIncrementSwitch','EngIdleDecrementSwitch','EngTestModeSwitch','EngShutdownOverrideSwitch'},'SgnStartBit',{0,2,4,6,8,24,26,28,30,32,34,36,38,40,48,53,56,58,60,62},'SgnLength',{2,2,2,2,16,2,2,2,2,2,2,2,2,8,5,3,2,2,2,2},'SgnType',{'standard','standard','standard','standard','standard','standard','standard','standard','standard','standard','standard','standard','standard','standard','standard','standard','standard','standard','standard','standard'},'ModeValue',{-1,-1,-1,-1,-1,-1,-1,-1,-1,-1,-1,-1,-1,-1,-1,-1,-1,-1,-1,-1},'DataType',{['unsigned int'],['unsigned int'],['unsigned int'],['unsigned int'],['unsigned int'],['unsigned int'],['unsigned int'],['unsigned int'],['unsigned int'],['unsigned int'],['unsigned int'],['unsigned int'],['unsigned int'],['unsigned int'],['unsigned int'],['unsigned int'],['unsigned int'],['unsigned int'],['unsigned int'],['unsigned int']},'ByteLayout',{['little endian'],['little endian'],['little endian'],['little endian'],['little endian'],['little endian'],['little endian'],['little endian'],['little endian'],['little endian'],['little endian'],['little endian'],['little endian'],['little endian'],['little endian'],['little endian'],['little endian'],['little endian'],['little endian'],['little endian']},'Factor',{1,1,1,1,2^-8,1,1,1,1,1,1,1,1,1,1,1,1,1,1,1},'Offset',{0,0,0,0,0,0,0,0,0,0,0,0,0,0,0,0,0,0,0,0},'SLDataType',{'SS_DOUBLE','SS_DOUBLE','SS_DOUBLE','SS_DOUBLE','SS_DOUBLE','SS_DOUBLE','SS_DOUBLE','SS_DOUBLE','SS_DOUBLE','SS_DOUBLE','SS_DOUBLE','SS_DOUBLE','SS_DOUBLE','SS_DOUBLE','SS_DOUBLE','SS_DOUBLE','SS_DOUBLE','SS_DOUBLE','SS_DOUBLE','SS_DOUBLE'}),'StatusSelected','yes','TimeSelected','yes','DeltaTimeSelected','yes','BytePortSelected','no','MessageLengthSelected','no','TriggerPort',struct('Selected','no','TriggerType',0),'UserCoding',struct('Selected','no','InterfaceFile','UserDecodingFile','FcnName','UserDecodeFcn','InportSelected','no','InportWidth',1,'OutportSelected','no','OutportWidth',1),'EnablePortSelected','yes','UseRXService','yes','BoardType','DS1','BoardNo',1,'ControllerNo',1),'OFF',[]}},'TLCFileName',{{'rtican_rx_message','OFF',[]}})  RTISFcnParameters=struct('SFcnRTICANMessage','struct','TLCFileName','char')  RTIBlockParaDefault=struct('BoardTypeNo',4302,'BoardNo',1,'ChannelNo',1,'Parameters',struct('DataFileSupport',struct('DataFileSelectedMaster',0,'DataFileSelectedLocal',0,'DataFileName','','DataFileDate','','SelectedFile',['<no file selected>']),'Options',struct('StatusSelected',1,'TimeSelected',1,'DeltaTimeSelected',1,'BytePortSelected',0,'MessageLengthSelected',0,'TriggerPort',struct('Selected',0,'TriggerType','rising'),'UserCoding',struct('Selected',0,'InterfaceFile','UserDecodingFile','FcnName','UserDecodeFcn','InportSelected',0,'InportWidth',1,'OutportSelected',0,'OutportWidth',1),'EnablePortSelected',0,'SignalOnPortnameSelected',1,'UseRXService',0),'Message',struct('MsgOnBlocknameSelected',0,'MsgName',['RX Message'],'MsgIdFormat',0,'MsgId',100,'MsgLength',8,'NumSignals',1,'SampleTime',-1,'Signal',struct('SgnName',['RX signal'],'SgnStartBit',0,'SgnLength',8,'SgnType',0,'ModeValue',-1,'DataType',0,'SLDataType','SS_DOUBLE','ByteLayout',0,'Factor',1,'Offset',0,'Min',0,'Max',255,'SgnComment',{{}},'SgnUnit',''),'MsgIdNumFormat',0,'MsgComment',{{''}}),'Version',1.2,'general',struct('isFromLib',1)),'GroupId',struct('Group',{{'RTICAN'}},'No',1,'Behavior',{{'NAMECHANGE'}},'BlockType',{{'SINK'}},'NameChangeFlag',0),'SFcnRTICANMessage',struct('MsgType','RX','MsgName',['RX Message'],'MsgIdFormat','STD','MsgId',100,'MsgLength',8,'NumSignals',1,'SampleTime',-1,'Signal',struct('SgnName',['RX signal'],'SgnStartBit',0,'SgnLength',8,'SgnType','standard','ModeValue',-1,'DataType',['unsigned int'],'ByteLayout',['little endian'],'SLDataType','SS_DOUBLE','Factor',1,'Offset',0),'StatusSelected','yes','TimeSelected','yes','DeltaTimeSelected','yes','BytePortSelected','no','MessageLengthSelected','no','EnablePortSelected','no','UserCoding',struct('Selected','no','InterfaceFile','UserDecodingFile','FcnName','UserDecodeFcn','InportSelected','no','InportWidth',1,'OutportSelected','no','OutportWidth',1),'TriggerPort',struct('Selected','no','TriggerType','rising'),'UseRXService','no','BoardType','DS4302','BoardNo',1,'ControllerNo',1,'SFcnPortType','Scalar'),'TLCFileName','rtican_rx_message')
      settings: AttributesFormatString=Group Id: RTICAN25\n  SourceProductName=dSPACE RTI CAN Blockset
  Data Type Conversion10 : DataTypeConversion  OutDataTypeStr=double  SaturateOnIntegerOverflow=on
  Data Type Conversion8 : DataTypeConversion  OutDataTypeStr=boolean  SaturateOnIntegerOverflow=on
  Data Type Conversion9 : DataTypeConversion  OutDataTypeStr=double  SaturateOnIntegerOverflow=on
  CCVS1_0 : Outport
  wires:
  CCVS1_00/5 -> Bus Creator/5  "WheelBasedVehicleSpeed"
  CCVS1_00/6 -> Bus Creator/6  "CruiseCtrlActive"
  CCVS1_00/4 -> Bus Creator/4  "ParkBrakeReleaseInhibitRq"
  CCVS1_00/3 -> Bus Creator/3  "CruiseCtrlPauseSwitch"
  CCVS1_00/1 -> Bus Creator/1  "TwoSpeedAxleSwitch"
  CCVS1_00/2 -> Bus Creator/2  "ParkingBrakeSwitch"
  CCVS1_00/17 -> Bus Creator/17  "EngIdleIncrementSwitch"
  CCVS1_00/18 -> Bus Creator/18  "EngIdleDecrementSwitch"
  CCVS1_00/19 -> Bus Creator/19  "EngTestModeSwitch"
  CCVS1_00/20 -> Bus Creator/20  "EngShutdownOverrideSwitch"
  CCVS1_00/7 -> Bus Creator/7  "CruiseCtrlEnableSwitch"
  CCVS1_00/10 -> Bus Creator/10  "CruiseCtrlSetSwitch"
  CCVS1_00/9 -> Bus Creator/9  "ClutchSwitch"
  CCVS1_00/8 -> Bus Creator/8  "BrakeSwitch"
  CCVS1_00/15 -> Bus Creator/15  "PTOGovernorState"
  CCVS1_00/14 -> Bus Creator/14  "CruiseCtrlSetSpeed"
  CCVS1_00/16 -> Bus Creator/16  "CruiseCtrlStates"
  CCVS1_00/11 -> Bus Creator/11  "CruiseCtrlCoastSwitch"
  CCVS1_00/12 -> Bus Creator/12  "CruiseCtrlResumeSwitch"
  CCVS1_00/13 -> Bus Creator/13  "CruiseCtrlAccelerateSwitch"
  Data Type Conversion9/1 -> Bus Creator3/3  "RX_time"
  Data Type Conversion10/1 -> Bus Creator3/4  "RX_delta_time"
  Data Type Conversion8/1 -> Bus Creator3/2  "RX_status"
  CCVS1_00/21 -> Data Type Conversion8/1
  CCVS1_00/22 -> Data Type Conversion9/1
  CCVS1_00/23 -> Data Type Conversion10/1
  Enable/1 -> CCVS1_00/Enable
  Bus Creator/1 -> Bus Creator3/1  "CCVS1Data"
  Bus Creator3/1 -> CCVS1_0/1  "CCVS1_E3"
